simulink model "robot_movil"  (R2015a)
settings: Solver=ode45  StartTime=0.0  StopTime=10.0  RelTol=1e-3
settings Model: Creator=rojas-j  LastModifiedBy=rojas-j

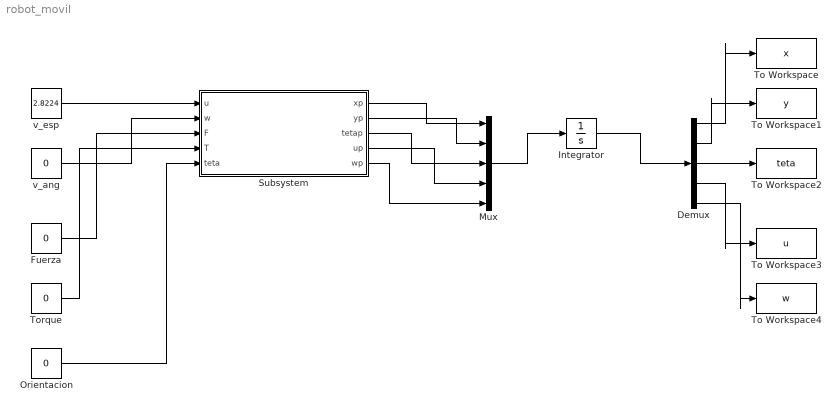
== system robot_movil ==
  Demux : Demux  Outputs=5
  Fuerza : Constant  Value=0
  Integrator : Integrator
  Mux : Mux  Inputs=5
  Orientacion : Constant  Value=0
  Subsystem : Subsystem
  To Workspace : ToWorkspace  VariableName=x  SaveFormat=Timeseries  SampleTime=-1
  To Workspace1 : ToWorkspace  VariableName=y  SaveFormat=Timeseries  SampleTime=-1
  To Workspace2 : ToWorkspace  VariableName=teta  SaveFormat=Timeseries  SampleTime=-1
  To Workspace3 : ToWorkspace  VariableName=u  SaveFormat=Timeseries  SampleTime=-1
  To Workspace4 : ToWorkspace  VariableName=w  SaveFormat=Timeseries  SampleTime=-1
  Torque : Constant  Value=0
  v_ang : Constant  Value=0
  v_esp : Constant  Value=2.8224
  wires:
  v_esp/1 -> Subsystem/1(u)
  v_ang/1 -> Subsystem/2(w)
  Fuerza/1 -> Subsystem/3(F)
  Torque/1 -> Subsystem/4(T)
  Orientacion/1 -> Subsystem/5(teta)
  Subsystem/1(xp) -> Mux/1
  Subsystem/2(yp) -> Mux/2
  Subsystem/3(tetap) -> Mux/3
  Subsystem/4(up) -> Mux/4
  Subsystem/5(wp) -> Mux/5
  Mux/1 -> Integrator/1
  Integrator/1 -> Demux/1
  Demux/1 -> To Workspace/1
  Demux/2 -> To Workspace1/1
  Demux/3 -> To Workspace2/1
  Demux/4 -> To Workspace3/1
  Demux/5 -> To Workspace4/1

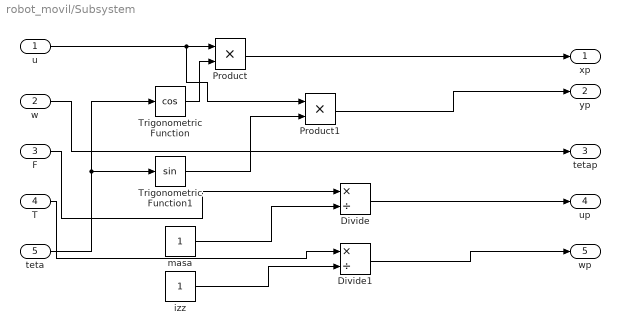
== system robot_movil/Subsystem ==
  u : Inport
  w : Inport  Port=2
  F : Inport  Port=3
  T : Inport  Port=4
  teta : Inport  Port=5
  Divide : Product  Inputs=*/
  Divide1 : Product  Inputs=*/
  Product : Product
  Product1 : Product
  Trigonometric Function : Trigonometry  Operator=cos
  Trigonometric Function1 : Trigonometry
  izz : Constant
  masa : Constant
  xp : Outport
  yp : Outport  Port=2
  tetap : Outport  Port=3
  up : Outport  Port=4
  wp : Outport  Port=5
  wires:
  u/1 -> Product/1, Product1/1
  Trigonometric Function/1 -> Product/2
  teta/1 -> Trigonometric Function1/1, Trigonometric Function/1
  Product/1 -> xp/1
  w/1 -> tetap/1
  F/1 -> Divide/1
  masa/1 -> Divide/2
  Divide/1 -> up/1
  izz/1 -> Divide1/2
  T/1 -> Divide1/1
  Divide1/1 -> wp/1
  Trigonometric Function1/1 -> Product1/2
  Product1/1 -> yp/1
